simulink model "kalman_filter1"  (Simulink 7.8)
settings: Solver=ode45  StartTime=0.0  StopTime=0.05  RelTol=1e-3
values from neighbouring files (symbols this model uses):
  fm = sqrt(f1*f2)    [band_sperr1.m]
  h = firpm(64,f,m)    [CFIR_1.m]    (also in adapt_filter1.m = adaptfilt.lms(ni,mu); adapt_filter2.m = adaptfilt.blms(ni,mu,1,36); adaptiv_2.m = [1 2 3 4 5 6 7 8 9 10]; adaptiv_3.m = [1 2 3 4 5 6 7 8 9 10])
  hr = 0.8.^(0:nf-1)    [block_lms_.m]
  Ts = 1/fs    (= 6.25e-05)    [G722_1.m]    (also in adaptiv_2.m = 0.001; adaptiv_3.m = 0.001; adaptiv_4.m = 0.001; adaptiv_5.m = 0.001)
undefined symbols (not defined in the file or in its folder): fst, get
libraries: dspobslib x1, dspstat3 x1, dspsnks4 x1
settings Model: Creator=svenhoffmann  LastModifiedBy=josef  ExtModeAutoUpdateStatusClock=off
settings DataIOCC: SignalLoggingName=sigsOut
settings DebuggingCC: SaveWithParameterizedLinksMsg=none  SignalResolutionControl=TryResolveAllWithWarning  SolverPrmCheckMsg=none  MultiTaskDSMMsg=warning  MultiTaskCondExecSysMsg=none  StrictBusMsg=None
settings HardwareCC: TargetUnknown=on
settings RTWCC: IncludeERTFirstTime=on

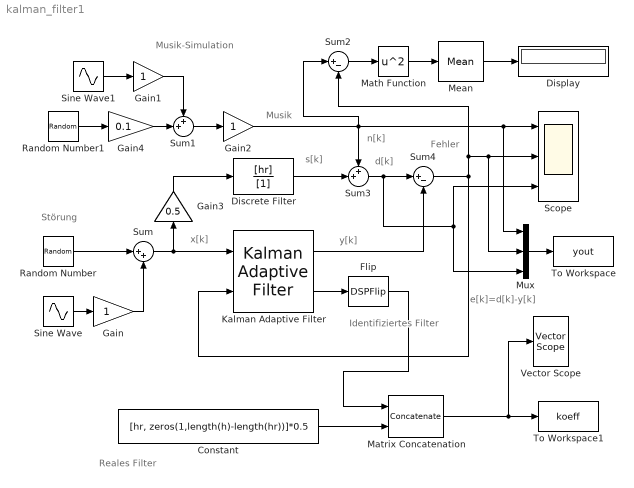
== system kalman_filter1 ==
  note: Musik
  note: Störung
  note: Musik-Simulation
  note: Fehler
  note: s[k]
  note: n[k]
  note: d[k]
  note: y[k]
  note: x[k]
  note: e[k]=d[k]-y[k]
  note: Reales Filter
  note: Identifiziertes Filter
  Constant : Constant  Value=[hr, zeros(1,length(h)-length(hr))]*0.5
  Discrete Filter : DiscreteFilter  Numerator=[hr]  Denominator=[1]  SampleTime=Ts
  Display : Display
  Flip : DSPFlip
  Gain : Gain  SaturateOnIntegerOverflow=on  OutDataTypeStr=Inherit: Same as input  ParamDataTypeStr=Inherit: Same as input
  Gain1 : Gain  SaturateOnIntegerOverflow=on  OutDataTypeStr=Inherit: Same as input  ParamDataTypeStr=Inherit: Same as input
  Gain2 : Gain  SaturateOnIntegerOverflow=on  OutDataTypeStr=Inherit: Same as input  ParamDataTypeStr=Inherit: Same as input
  Gain3 : Gain  Gain=0.5  SaturateOnIntegerOverflow=on  OutDataTypeStr=Inherit: Same as input  ParamDataTypeStr=Inherit: Same as input
  Gain4 : Gain  Gain=0.1  SaturateOnIntegerOverflow=on  OutDataTypeStr=Inherit: Same as input  ParamDataTypeStr=Inherit: Same as input
  Kalman Adaptive Filter : dspobslib/Kalman Adaptive Filter  Ntaps=M  Jmin=QM  q=0  ic0=0  K0=0.5  Adapt=off  RstPort=None
  Math Function : Math  Operator=square  SaturateOnIntegerOverflow=on
  Matrix Concatenation : Concatenate  Mode=Multidimensional array  ConcatenateDimension=2
  Mean : dspstat3/Mean  run=on  reset_popup=None  InputProcessing=Inherited (this choice will be removed - see release notes)  directionMode=Each column  dimension=1  treatSBRowAsCol=on  roiEnable=off  roiType=Rectangles  roiPortion=Entire ROI  roiOutput=Individual statistics for each ROI  roiFlag=off  outputDataTypeStr=Inherit: Same as accumulator  outputLastDataTypeStr=Inherit: Same as accumulator  outputMin=[]  outputMax=[]  roundingMode=Floor  overflowMode=off
  Mux : Mux  Inputs=3
  Random Number : RandomNumber  SampleTime=Ts
  Random Number1 : RandomNumber  Seed=1739  SampleTime=Ts
  Scope : Scope  NumInputPorts=3
      settings: YMin=-2~-5~-5  YMax=2~5~5
  Sine Wave : Sin  Frequency=2*pi*fst  SampleTime=Ts
  Sine Wave1 : Sin  Frequency=2*pi*fm  SampleTime=Ts
  Sum : Sum  Inputs=|++  SaturateOnIntegerOverflow=on
  Sum1 : Sum  Inputs=++|  SaturateOnIntegerOverflow=on
  Sum2 : Sum  Inputs=|+-  SaturateOnIntegerOverflow=on
  Sum3 : Sum  Inputs=++|  SaturateOnIntegerOverflow=on
  Sum4 : Sum  Inputs=|+-  SaturateOnIntegerOverflow=on
  To Workspace : ToWorkspace  VariableName=yout  SampleTime=-1  SaveFormat=Structure With Time
  To Workspace1 : ToWorkspace  VariableName=koeff  SampleTime=-1  SaveFormat=Structure
      settings: Decimation=100
  Vector Scope : dspsnks4/Vector Scope  ScopeProperties=off  Domain=Time  HorizSpan=1  DisplayProperties=off  AxisGrid=on  Memory=off  FrameNumber=on  AxisLegend=off  AxisZoom=off  OpenScopeAtSimStart=on  OpenScopeImmediately=off  FigPos=get(0,'defaultfigureposition')  AxisProperties=off  XUnits=Hertz  XRange=[0...Fs/2]  InheritXIncr=on  XIncr=1  XLabel=Time  XLimit=Auto  XMin=0  XMax=1  XStart=0  YUnits=dB  YLabel=Amplitude  LineProperties=on  LineMarkers=*  XAxisParamsVer=6.8
      settings: YMin=-0.0303642523190484  YMax=0.233455043343824
  wires:
  Sine Wave/1 -> Gain/1
  Random Number/1 -> Sum/1
  Gain/1 -> Sum/2
  Sum/1 -> Gain3/1, Kalman Adaptive Filter/1
  Sine Wave1/1 -> Gain1/1
  Discrete Filter/1 -> Sum3/2
  Constant/1 -> Matrix Concatenation/2
  Matrix Concatenation/1 -> Vector Scope/1, To Workspace1/1
  Sum1/1 -> Gain2/1
  Sum3/1 -> Sum4/1, Scope/3, Mux/3
  Sum4/1 -> Sum2/2, Scope/2, Mux/2, Kalman Adaptive Filter/2
  Kalman Adaptive Filter/1 -> Sum4/2
  Random Number1/1 -> Gain4/1
  Gain1/1 -> Sum1/1
  Gain2/1 -> Sum3/1, Sum2/1, Scope/1, Mux/1
  Gain3/1 -> Discrete Filter/1
  Gain4/1 -> Sum1/2
  Sum2/1 -> Math Function/1
  Math Function/1 -> Mean/1
  Mean/1 -> Display/1
  Mux/1 -> To Workspace/1
  Kalman Adaptive Filter/2 -> Flip/1
  Flip/1 -> Matrix Concatenation/1
